simulink model "Neutron_f"  (Simulink 7.9)
settings: Solver=ode45  StartTime=0.0  StopTime=10.0  RelTol=1e-3
values from neighbouring files (symbols this model uses):
  a = -1.0    (= -1)    [parameters.m]
  b = -2.0    (= -2)    [parameters.m]
  c = 0.23    [parameters.m]
  Ta = 0.38    [parameters.m]
  Tr = 0.04    [parameters.m]
settings Model: Creator=dede  LastModifiedBy=dede

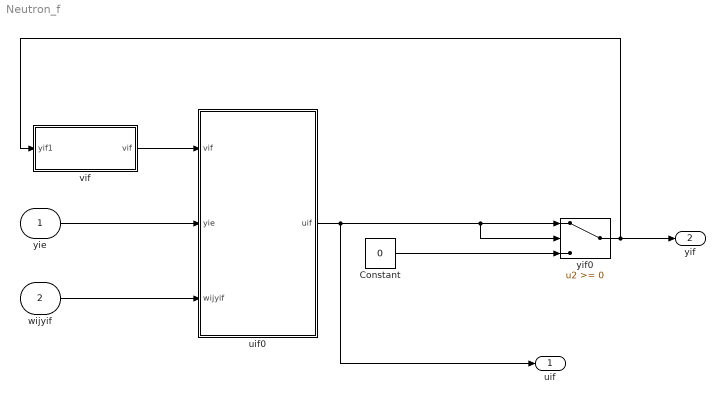
== system Neutron_f ==
  yie : Inport
  wijyif : Inport  Port=2
  Constant : Constant  Value=0
  uif0 : Subsystem
  vif : Subsystem
  yif0 : Switch
  uif : Outport
  yif : Outport  Port=2
  wires:
  vif/1(vif) -> uif0/1(vif)
  Constant/1 -> yif0/3
  uif0/1(uif) -> yif0/1, yif0/2, uif/1
  yif0/1 -> vif/1(yif1), yif/1
  yie/1 -> uif0/2(yie)
  wijyif/1 -> uif0/3(wijyif)

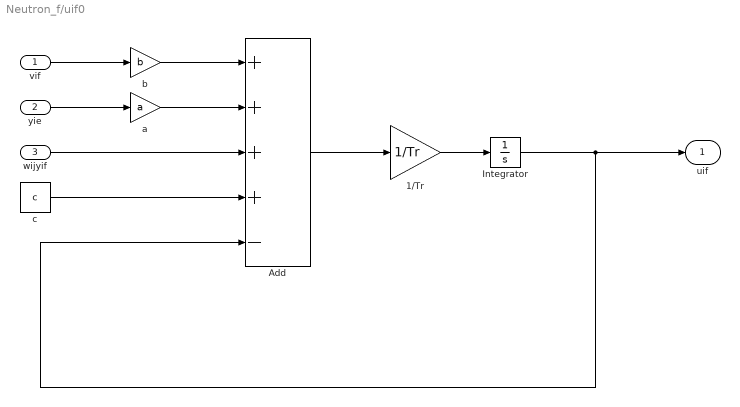
== system Neutron_f/uif0 ==
  vif : Inport
  yie : Inport  Port=2
  wijyif : Inport  Port=3
  1/Tr : Gain  Gain=1/Tr
  Add : Sum  Inputs=++++-
  Integrator : Integrator
  a : Gain  Gain=a
  b : Gain  Gain=b
  c : Constant  Value=c
  uif : Outport
  wires:
  vif/1 -> b/1
  b/1 -> Add/1
  yie/1 -> a/1
  a/1 -> Add/2
  wijyif/1 -> Add/3
  c/1 -> Add/4
  Add/1 -> 1/Tr/1
  1/Tr/1 -> Integrator/1
  Integrator/1 -> Add/5, uif/1

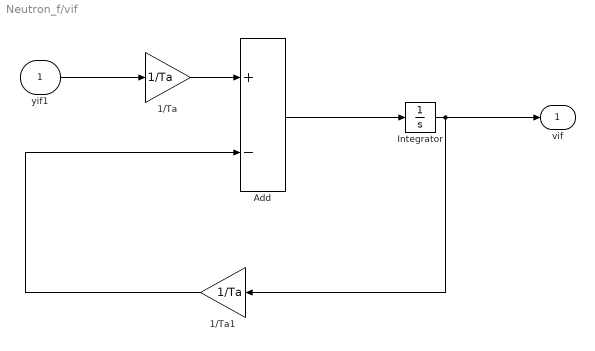
== system Neutron_f/vif ==
  yif1 : Inport
  1/Ta : Gain  Gain=1/Ta
  1/Ta1 : Gain  Gain=1/Ta
  Add : Sum  Inputs=+-
  Integrator : Integrator
  vif : Outport
  wires:
  yif1/1 -> 1/Ta/1
  1/Ta/1 -> Add/1
  Add/1 -> Integrator/1
  Integrator/1 -> 1/Ta1/1, vif/1
  1/Ta1/1 -> Add/2
